simulink model "PubIfDecisionLSM_MDL"  (R2020b)
settings: configuration reference "DspaceConfig" (kept outside this file)
PostLoadFcn:
  | if any(exist('dsrtsu_mdlpostloadfcn', 'file') ~= 0), dsrtsu_mdlpostloadfcn('Execute', bdroot); end
InitFcn:
  | , if any(exist('rtifpga_mdlclblib', 'file') ~= 0), rtifpga_mdlclblib('Init', bdroot); end,
  | , if any(exist('dsmpb_private', 'file') ~= 0), dsmpb_private('dsmpb_mdlclblib', 'Init', bdroot); end,
values from neighbouring files (symbols this model uses):
  P_LSM_ALC_Enable = 0.0    [LSM_Parameter.sldd]
  P_LSM_AwayEdge_offset = 0.1    [LSM_Parameter.sldd]
  P_LSM_CentValidErr = 1.0    [LSM_Parameter.sldd]
  P_LSM_DOP_C0_EN_Limit = 0.8    [LSM_Parameter.sldd]
  P_LSM_DOP_C0_out_Limit = 2.0    [LSM_Parameter.sldd]
  P_LSM_DOP_C1_EN_Limit : value not decoded    [LSM_Parameter.sldd]
  P_LSM_DOP_C1_out_Limit : value not decoded    [LSM_Parameter.sldd]
  P_LSM_DOP_C1AndC2_Lim_X : value not decoded    [LSM_Parameter.sldd]
  P_LSM_DOP_C2_EN_Limit : value not decoded    [LSM_Parameter.sldd]
  P_LSM_DOP_C2_out_Limit : value not decoded    [LSM_Parameter.sldd]
  P_LSM_DOP_In_Pre2Dop_Dis = 1.0    [LSM_Parameter.sldd]
  P_LSM_DOP_Out_Pre2Dop_Dis = 2.0    [LSM_Parameter.sldd]
  P_LSM_DOP_PreDis_X : value not decoded    [LSM_Parameter.sldd]
  P_LSM_DOP_PreDis_Y : value not decoded    [LSM_Parameter.sldd]
  P_LSM_DOPEnableSW = 1.0    [LSM_Parameter.sldd]
  P_LSM_DOPValid_CheckTime = 0.06    [LSM_Parameter.sldd]
  P_LSM_DoubleLine_Curr2Cent_Dislimit = 0.5    [LSM_Parameter.sldd]
  P_LSM_DoubleLine_Dop2Cent_Dislimit = 0.5    [LSM_Parameter.sldd]
  P_LSM_DoubleLine_DOPOut_C1 : value not decoded    [LSM_Parameter.sldd]
  P_LSM_DoubleLine_Pre2Cent_Dislimit = 1.0    [LSM_Parameter.sldd]
  P_LSM_Error_Limit = 0.5    [LSM_Parameter.sldd]
  P_LSM_IFV2CenterAxis = 0.0    [LSM_Parameter.sldd]
  P_LSM_IFV2RearAxis = 0.0    [LSM_Parameter.sldd]
  P_LSM_Line2Edge_limit = 0.5    [LSM_Parameter.sldd]
  P_LSM_Line_Error = 0.1    [LSM_Parameter.sldd]
  P_LSM_LineSTD_Limit = 0.15    [LSM_Parameter.sldd]
  P_LSM_NOH_Switch = 0.0    [LSM_Parameter.sldd]
  P_LSM_OTL_C0_Factor = 1.0    [LSM_Parameter.sldd]
  P_LSM_OTL_C1_Factor = 0.5    [LSM_Parameter.sldd]
  P_LSM_OTL_C2_Factor = 0.5    [LSM_Parameter.sldd]
  P_LSM_Pre2OnlyLineDis = 5.0    [LSM_Parameter.sldd]
  P_LSM_Pre_t = 0.0    [LSM_Parameter.sldd]
  P_LSM_SingleLine_Cent2Edge_Dislimit = 100.0    [LSM_Parameter.sldd]
  P_LSM_SingleLine_Curr2Cent_Dislimit = 0.2    [LSM_Parameter.sldd]
  P_LSM_SingleLine_Dop2Cent_Dislimit = 0.2    [LSM_Parameter.sldd]
  P_LSM_SingleLine_DOPOut_C1 : value not decoded    [LSM_Parameter.sldd]
  P_LSM_SingleLine_Pre2Cent_Dislimit = 0.5    [LSM_Parameter.sldd]
  P_LSM_TJALimitSpd = 60.0    [LSM_Parameter.sldd]
undefined symbols (not defined in the file or in its folder): P_lCS_IFV2CenterAxis, P_LCS_IFV2RearAxis, P_LSM_EntryEdge_offset, P_LSM_EntryLnChngEnSwitch, P_LSM_EntryVanishDis, P_LSM_LinetLostTime, P_LSM_LineWijCal_C12, P_LSM_LineWijCal_C13, P_LSM_MapValid_ErrorSwitch, P_LSM_PosLineLcFac, P_LSM_SpdLim_Stub_Spd, P_LSM_SpdLim_StubLength, P_LSM_SpdTurnAlarm
libraries: simulink x324, TrueDurationTime x11
(part 12 of 25)

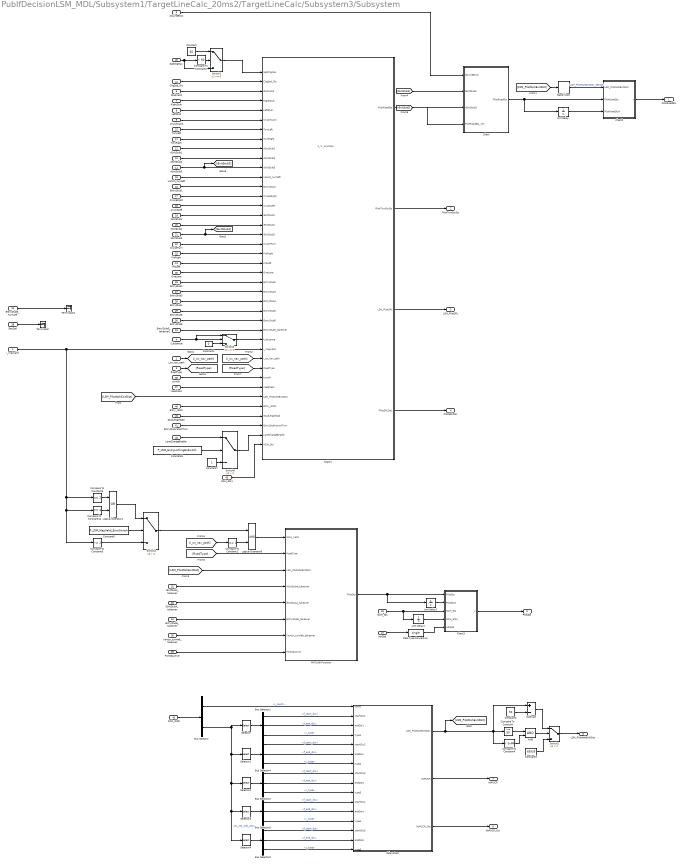
== system PubIfDecisionLSM_MDL/Subsystem1/TargetLineCalc_20ms2/TargetLineCalc/Subsystem3/Subsystem ==
  note: b_is_available
  i_mapvalid : Inport
  i_on_nav_path : Inport  Port=2
  RoadType : Inport  Port=3
  f_distance : Inport  Port=4
  bIsLineExist : Inport  Port=5
  StubValid : Inport  Port=6
  RightStub : Inport  Port=7
  LeftStub : Inport  Port=8
  CruiseValid : Inport  Port=9
  TurnLeft : Inport  Port=10
  TurnRight : Inport  Port=11
  rExitStub1 : Inport  Port=12
  rExitStub2 : Inport  Port=13
  rExitStub3 : Inport  Port=14
  Vanish_turnleft : Inport  Port=15
  EntryStub1 : Inport  Port=16
  CruiseRight : Inport  Port=17
  CruiseLeft : Inport  Port=18
  lExitStub1 : Inport  Port=19
  lExitStub2 : Inport  Port=20
  lExitStub3 : Inport  Port=21
  CruiseTurn : Inport  Port=22
  FrbRight : Inport  Port=23
  FrbLeft : Inport  Port=24
  OneLane : Inport  Port=25
  EntryStub2 : Inport  Port=26
  EntryStub3 : Inport  Port=27
  EntryStub4 : Inport  Port=28
  EntryStub5 : Inport  Port=29
  EntryStub6 : Inport  Port=30
  EntryStub5_TurnLeft : Inport  Port=31
  rExitStub4_takeover : Inport  Port=32
  lExitStub4_takeover : Inport  Port=33
  EntryStub5_takeover : Inport  Port=34
  Vanish_turnleft_takeover : Inport  Port=35
  turndir : Inport  Port=36
  roadClass : Inport  Port=37
  DecSpd : Inport  Port=38  OutDataTypeStr=uint8
  ForbidActive : Inport  Port=39
  StudLengthSpd : Inport  Port=40
  EntryStubVanishTurn : Inport  Port=41
  RFM_ODD : Inport  Port=42  OutDataTypeStr=Bus: RFM_ODD_BUS  PortDimensions=1  BusOutputAsStruct=on
  NOH_Sts : Inport  Port=43
  ChgSpd_Dis : Inport  Port=44
  SpdChgMax : Inport  Port=45
  Entry_dC0V : Inport  Port=46
  vehSpd : Inport  Port=47
  LaneChangeEnable : Inport  Port=48
  AND : Logic  AllPortsSameDT=off  OutDataTypeStr=boolean
  Bus Selector : BusSelector  OutputSignals=i_count,st_not_odd_vec
  Bus Selector{1..5} (5 alike) : BusSelector  OutputSignals=f_start_dis,f_end_dis,i_type
  Chart : Stateflow chart  TreatAsAtomicUnit=on
      settings: PortSchema="{\"entries\":[{\"content\":{\"sides\":[{\"content\":{\"connectorIds\":[\"In2\",\"In3\",\"In4\",\"In1\"]},\"type\":\"ConnectorPlacement.EquallySpacedRectSide\",\"uuid\":\"cb5dbf47-71a9-4c68-a9a0-e20b9a6c2f96\"},{\"content\":{\"connectorIds\":[\"Out1\"],\"side\":\"RIGHT\"},\"type\":\"ConnectorPlacement.EquallySpacedRectSide\",\"uuid\":\"d94cb245-01e7-4aac-95f6-b5a2c86f74a4\"},{\"content\":{\"connectorIds\":[],\"side\":\"TOP\"},\"type\":\"ConnectorPlacement.EquallySpacedRectSide\",\"uuid\":\"b16bae50-db94-4c56-a3f9-d57c33f49c97\"},{\"content\":{\"connectorIds\":[],\"side\":\"HIDDEN\"},\"type\":\"ConnectorPlacement.EquallySpacedRectSide\",\"uuid\":\"ebc0363f-4109-4233-98c7-946dda5a9c96\"}]},\"type\":\"ConnectorPlacement.EquallySpacedConnector\",\"uuid\":\"99392276-8e03-4fff-8aa1-93f14ecf3ea7\"}],\"packageUris\":[\"http://schema.mathworks.com/mf0/Connector/R2020b\"],\"version\":\"1.0\"}"
  Chart1 : Stateflow chart  TreatAsAtomicUnit=on
      settings: PortSchema="{\"entries\":[{\"content\":{\"sides\":[{\"content\":{\"connectorIds\":[\"In40\",\"In39\",\"In1\",\"In2\",\"In4\",\"In5\",\"In6\",\"In7\",\"In10\",\"In11\",\"In22\",\"In8\",\"In9\",\"In15\",\"In14\",\"In19\",\"In20\",\"In21\",\"In17\",\"In24\",\"In23\",\"In25\",\"In18\",\"In26\",\"In27\",\"In28\",\"In29\",\"In30\",\"In16\",\"In12\",\"In13\",\"In3\",\"In31\",\"In32\",\"In33\",\"In34\",\"In35\",\"In36\",\"In37\",\"In38\"]},\"type\":\"ConnectorPlacement.EquallySpacedRectSide\",\"uuid\":\"77f3efae-110f-49ea-917e-ae218e9f5cc2\"},{\"content\":{\"connectorIds\":[\"Out1\",\"Out2\",\"Out3\",\"Out4\"],\"side\":\"RIGHT\"},\"type\":\"ConnectorPlacement.EquallySpacedRectSide\",\"uuid\":\"2d94deb3-5275-495d-8df1-e01272a631f4\"},{\"content\":{\"connectorIds\":[],\"side\":\"TOP\"},\"type\":\"ConnectorPlacement.EquallySpacedRectSide\",\"uuid\":\"28314d3e-7dbf-498a-8d7e-47e3fdfafbd6\"},{\"content\":{\"connectorIds\":[],\"side\":\"HIDDEN\"},\"type\":\"ConnectorPlacement.EquallySpacedRectSide\",\"uuid\":\"3f9bf8b9-b1e2-405d-95be-6477a1260bee\"}]},\"type\":\"ConnectorPlacement.EquallySpacedConnector\",\"uuid\":\"276e7b9f-5b1f-44bf-bcdb-8855a9c8dee8\"}],\"packageUris\":[\"http://schema.mathworks.com/mf0/Connector/R2020b\"],\"version\":\"1.0\"}"
  Chart2 : Stateflow chart  TreatAsAtomicUnit=on
  Chart3 : Stateflow chart  TreatAsAtomicUnit=on
      settings: PortSchema="{\"entries\":[{\"content\":{\"sides\":[{\"content\":{\"connectorIds\":[\"In1\",\"In4\",\"In2\",\"In3\",\"In5\"]},\"type\":\"ConnectorPlacement.EquallySpacedRectSide\",\"uuid\":\"2a855711-103d-4afd-b0dc-20bc03fcd3b0\"},{\"content\":{\"connectorIds\":[\"Out1\"],\"side\":\"RIGHT\"},\"type\":\"ConnectorPlacement.EquallySpacedRectSide\",\"uuid\":\"9c6efe1d-7b4b-42ad-a8c7-d9bdd5462576\"},{\"content\":{\"connectorIds\":[],\"side\":\"TOP\"},\"type\":\"ConnectorPlacement.EquallySpacedRectSide\",\"uuid\":\"89e81c27-b573-4513-8c47-d8079b6a1114\"},{\"content\":{\"connectorIds\":[],\"side\":\"HIDDEN\"},\"type\":\"ConnectorPlacement.EquallySpacedRectSide\",\"uuid\":\"aa56bddb-9370-4270-a964-1a71b37db55c\"}]},\"type\":\"ConnectorPlacement.EquallySpacedConnector\",\"uuid\":\"d90e930b-4b5f-4761-8d41-dad0e7596f83\"}],\"packageUris\":[\"http://schema.mathworks.com/mf0/Connector/R2020b\"],\"version\":\"1.0\"}"
  Compare To Constant : simulink/Logic and Bit Operations/Compare To Constant  relop=>=  const=50  OutDataTypeStr=boolean
  Compare To Constant1 : simulink/Logic and Bit Operations/Compare To Constant  relop===  const=1  OutDataTypeStr=boolean
  Compare To Constant12 : simulink/Logic and Bit Operations/Compare To Constant  relop===  const=3  OutDataTypeStr=boolean
  Compare To Constant2 : simulink/Logic and Bit Operations/Compare To Constant  relop=<  const=60  OutDataTypeStr=boolean
  Compare To Constant4 : simulink/Logic and Bit Operations/Compare To Constant  relop=<  const=0xffff  OutDataTypeStr=boolean
  Compare To Constant5 : simulink/Logic and Bit Operations/Compare To Constant  relop===  const=2  OutDataTypeStr=boolean
  Compare To Constant6 : simulink/Logic and Bit Operations/Compare To Constant  relop=>=  const=2  OutDataTypeStr=boolean
  Constant : Constant  Value=60
  Constant2 : Constant  Value=50  OutDataTypeStr=uint16
  Constant3 : Constant  Value=65535  OutDataTypeStr=uint16
  Constant4 : Constant  Value=0  OutDataTypeStr=single
  Constant5 : Constant  Value=P_LSM_MapValid_ErrorSwitch
  Constant6 : Constant  Value=P_LSM_EntryLnChngEnSwitch
  Constant7 : Constant
  Data Type Conversion : DataTypeConversion  OutDataTypeStr=single
  EntryStub5_takeover1 : InportShadow  Port=34
  Logical Operator1 : Logic  Operator=OR  AllPortsSameDT=off  OutDataTypeStr=boolean
  Logical Operator6 : Logic  AllPortsSameDT=off  OutDataTypeStr=boolean
  MATLAB Function : MATLAB Function  TreatAsAtomicUnit=on
  NOH_Sts1 : InportShadow  Port=43
  Selector : Selector  InputPortWidth=5  IndexOptions=Index vector (dialog)  Indices=1  OutputSizes=1
  Selector1 : Selector  InputPortWidth=5  IndexOptions=Index vector (dialog)  Indices=2  OutputSizes=1
  Selector2 : Selector  InputPortWidth=5  IndexOptions=Index vector (dialog)  Indices=3  OutputSizes=1
  Selector3 : Selector  InputPortWidth=5  IndexOptions=Index vector (dialog)  Indices=4  OutputSizes=1
  Selector4 : Selector  InputPortWidth=5  IndexOptions=Index vector (dialog)  Indices=5  OutputSizes=1
  Signal Copy : SignalConversion  OverrideOpt=off
  Subsystem : Subsystem
  Subtract : Sum  Inputs=+-
  Switch1 : Switch
  Switch2 : Switch  Criteria=u2 > Threshold
  Switch3 : Switch
  Switch4 : Switch  Criteria=u2 > Threshold
  Switch6 : Switch  Criteria=u2 > Threshold
  Terminator : Terminator
  Terminator1 : Terminator
  Unit Delay : UnitDelay  SampleTime=-1  HasFrameUpgradeWarning=on
  Unit Delay1 : UnitDelay  SampleTime=-1  HasFrameUpgradeWarning=on
  Unit Delay2 : UnitDelay  SampleTime=-1  HasFrameUpgradeWarning=on
  PilotRoadSts : Outport
  PilotTurnSwSts : Outport  Port=2
  LSM_PilotSPL : Outport  Port=3
  PilotSPLDist : Outport  Port=4
  PilotSts : Outport  Port=5
  LSM_PilotNohExitDist : Outport  Port=6  OutDataTypeStr=uint16  PortDimensions=1  BusOutputAsStruct=on
  NoPUCR : Outport  Port=7
  NoPUCR_Dis : Outport  Port=8
  wires:
  ChgSpd_Dis/1 -> Chart1/39(ChgSpd_Dis)
  Switch1/1 -> Chart1/40(SpdChgMax)
  Constant/1 -> Switch1/1
  Compare To Constant2/1 -> Switch1/2
  SpdChgMax/1 -> Compare To Constant2/1, Switch1/3
  NOH_Sts1/1 -> Chart1/38(NOH_Sts)
  EntryStub5_takeover1/1 -> Chart1/30(EntryStub5_takeover)
  EntryStub5_TurnLeft/1 -> Terminator1/1
  Switch6/1 -> Chart1/37(LaneChangeEnable)
  EntryStubVanishTurn/1 -> Chart1/36(EntryStubVanishTurn)
  [RoadType] -> MATLAB Function/2(RoadType)
  [RoadType] -> Chart1/3(RoadType)
  RoadType/1 -> [RoadType]
  [i_on_nav_path] -> Compare To Constant1/1
  i_on_nav_path/1 -> [i_on_nav_path]
  Constant7/1 -> Switch6/3
  LaneChangeEnable/1 -> Switch6/1
  Constant6/1 -> Switch6/2
  Compare To Constant6/1 -> Switch4/3
  Switch4/1 -> Logical Operator6/1
  Constant5/1 -> Switch4/2
  Logical Operator1/1 -> Switch4/1
  Compare To Constant5/1 -> Logical Operator1/1
  Switch3/1 -> Chart1/16(f_distance)
  Constant4/1 -> Switch3/3
  Data Type Conversion/1 -> Chart3/5(vehSpd)
  Chart3/1(y) -> PilotSts/1
  StudLengthSpd/1 -> Chart1/35(StudLengthSpd)
  vehSpd/1 -> Data Type Conversion/1
  Unit Delay2/1 -> Chart3/4(PilotStsK)
  ForbidActive/1 -> MATLAB Function/8(ForbidActive)
  DecSpd/1 -> Terminator/1
  Subsystem/2(NoPUCR) -> NoPUCR/1
  Subsystem/3(NoPUCR_Dis) -> NoPUCR_Dis/1
  roadClass/1 -> Chart1/32(roadClass)
  Subsystem/1(LSM_PilotNohExitDist) -> [LSM_PilotNohExitDist], Compare To Constant4/1, Compare To Constant/1, Subtract/1
  Bus Selector3/3 -> Subsystem/16(type5)  "<i_type>"
  Bus Selector3/2 -> Subsystem/15(endDis5)  "<f_end_dis>"
  Bus Selector3/1 -> Subsystem/14(startDis5)  "<f_start_dis>"
  Bus Selector5/3 -> Subsystem/13(type4)  "<i_type>"
  Bus Selector5/2 -> Subsystem/12(endDis4)  "<f_end_dis>"
  Bus Selector5/1 -> Subsystem/11(startDis4)  "<f_start_dis>"
  Selector3/1 -> Bus Selector5/1
  Bus Selector2/3 -> Subsystem/10(type3)  "<i_type>"
  Bus Selector2/2 -> Subsystem/9(endDis3)  "<f_end_dis>"
  Bus Selector2/1 -> Subsystem/8(startDis3)  "<f_start_dis>"
  Bus Selector4/3 -> Subsystem/7(type2)  "<i_type>"
  Bus Selector4/2 -> Subsystem/6(endDis2)  "<f_end_dis>"
  Bus Selector1/3 -> Subsystem/4(type1)  "<i_type>"
  Bus Selector4/1 -> Subsystem/5(startDis2)  "<f_start_dis>"
  Bus Selector1/2 -> Subsystem/3(endDis1)  "<f_end_dis>"
  Bus Selector1/1 -> Subsystem/2(startDis1)  "<f_start_dis>"
  Bus Selector/1 -> Subsystem/1(count)  "<i_count>"
  Selector1/1 -> Bus Selector4/1
  Selector4/1 -> Bus Selector3/1
  Selector2/1 -> Bus Selector2/1
  Selector/1 -> Bus Selector1/1
  Bus Selector/2 -> Selector/1, Selector1/1, Selector2/1, Selector3/1, Selector4/1  "<st_not_odd_vec>"
  RFM_ODD/1 -> Bus Selector/1
  turndir/1 -> Chart1/31(turndir)
  f_distance/1 -> Switch3/2, Switch3/1
  Vanish_turnleft_takeover/1 -> MATLAB Function/7(Vanish_turnleft_takeover)
  EntryStub5_takeover/1 -> MATLAB Function/6(EntryStub5_takeover)
  lExitStub4_takeover/1 -> MATLAB Function/5(lExitStub4_takeover)
  rExitStub4_takeover/1 -> MATLAB Function/4(rExitStub4_takeover)
  i_mapvalid/1 -> Compare To Constant5/1, Compare To Constant6/1, Compare To Constant12/1, Chart1/12(i_mapvalid)
  Logical Operator6/1 -> MATLAB Function/1(NOH_Valid)
  MATLAB Function/1(PilotSts) -> Unit Delay2/1, Chart3/1(PilotSts)
  Compare To Constant1/1 -> Logical Operator6/2
  Compare To Constant12/1 -> Logical Operator1/2
  EntryStub2/1 -> Chart1/18(EntryStub2)
  [i_on_nav_path] -> Chart1/13(i_on_nav_path)
  lExitStub2/1 -> Chart1/20(lExitStub2)
  TurnRight/1 -> Chart1/7(TurnRight)
  rExitStub3/1 -> Chart1/22(rExitStub3), [rExitStub3]
  Chart1/4(PilotSPLDist) -> PilotSPLDist/1
  CruiseTurn/1 -> Chart1/17(CruiseTurn)
  StubValid/1 -> Chart1/1(StubValid)
  CruiseLeft/1 -> Chart1/14(CruiseLeft)
  EntryStub4/1 -> Chart1/27(EntryStub4)
  EntryStub3/1 -> Chart1/26(EntryStub3)
  OneLane/1 -> Chart1/25(OneLane)
  FrbLeft/1 -> Chart1/23(FrbLeft)
  CruiseRight/1 -> Chart1/15(CruiseRight)
  Vanish_turnleft/1 -> Chart1/8(Vanish_turnleft)
  LeftStub/1 -> Chart1/4(LeftStub)
  RightStub/1 -> Chart1/2(RightStub)
  lExitStub1/1 -> Chart1/19(lExitStub1)
  EntryStub6/1 -> Chart1/29(EntryStub6)
  bIsLineExist/1 -> Chart/2(bIsLineExist)
  CruiseValid/1 -> Chart1/5(CruiseValid)
  rExitStub1/1 -> Chart1/10(rExitStub1)
  Chart/1(PilotRoadSts) -> Chart2/2(PilotRoadSts), Unit Delay/1
  EntryStub1/1 -> Chart1/9(EntryStub1)
  rExitStub2/1 -> Chart1/11(rExitStub2)
  TurnLeft/1 -> Chart1/6(TurnLeft)
  [lExitStub3] -> Chart/3(lExitStub3)
  Chart1/1(PilotRoadSts) -> Chart/1(PilotRoadSts_init)
  FrbRight/1 -> Chart1/24(FrbRight)
  EntryStub5/1 -> Chart1/28(EntryStub5)
  lExitStub3/1 -> Chart1/21(lExitStub3), [lExitStub3]
  [rExitStub3] -> Chart/4(rExitStub3)
  Chart1/2(PilotTurnSwSts) -> PilotTurnSwSts/1
  [LSM_PilotNohExitDist] -> Chart1/33(LSM_PilotNohExitDist)
  Chart2/1(y) -> PilotRoadSts/1
  Unit Delay/1 -> Chart2/3(PilotRoadStsK)
  [LSM_PilotNohExitDist] -> Signal Copy/1
  Signal Copy/1 -> Chart2/1(LSM_PilotNohExitDist)  "LSM_PilotNohExitDist_Set100"
  NOH_Sts/1 -> Unit Delay1/1, Chart3/2(NOH_Sts)
  Unit Delay1/1 -> Chart3/3(NOH_StsK)
  [LSM_PilotNohExitDist] -> MATLAB Function/3(LSM_PilotNohExitDist)
  Entry_dC0V/1 -> Chart1/34(Entry_dC0V)
  Chart1/3(LSM_PilotSPL) -> LSM_PilotSPL/1
  Constant2/1 -> Subtract/2
  Switch2/1 -> LSM_PilotNohExitDist/1
  Compare To Constant/1 -> AND/1
  Subtract/1 -> Switch2/1
  Constant3/1 -> Switch2/3
  Compare To Constant4/1 -> AND/2
  AND/1 -> Switch2/2

== system PubIfDecisionLSM_MDL/Subsystem1/TargetLineCalc_20ms2/TargetLineCalc/Subsystem3/Subsystem1 ==
  i_mapvalid : Inport
  i_on_nav_path : Inport  Port=2
  RoadType : Inport  Port=3
  NoPUCR : Inport  Port=4
  f_distance : Inport  Port=5
  MATLAB Function : MATLAB Function  TreatAsAtomicUnit=on
  Subsystem : Subsystem
  Unit Delay{,1..9} (10 alike) : UnitDelay  SampleTime=-1  HasFrameUpgradeWarning=on
  i_mapvalid_out : Outport
  i_on_nav_path_out : Outport  Port=2
  RoadType_out : Outport  Port=3
  wires:
  NoPUCR/1 -> Subsystem/2(NoPUCR)
  MATLAB Function/3(RoadType_out) -> RoadType_out/1
  Unit Delay9/1 -> MATLAB Function/7(f_distanceK)
  Unit Delay8/1 -> MATLAB Function/6(RoadTypeK)
  Unit Delay6/1 -> MATLAB Function/4(i_on_nav_pathK)
  Unit Delay5/1 -> MATLAB Function/2(i_mapvalidK)
  i_mapvalid/1 -> MATLAB Function/1(i_mapvalid), Unit Delay5/1
  RoadType/1 -> MATLAB Function/5(RoadType), Unit Delay8/1
  i_on_nav_path/1 -> MATLAB Function/3(i_on_nav_path), Unit Delay6/1
  f_distance/1 -> Unit Delay9/1
  Unit Delay/1 -> MATLAB Function/12(i_on_nav_path_storeK)
  MATLAB Function/6(RoadStore) -> Unit Delay2/1
  MATLAB Function/4(count) -> Unit Delay4/1
  Unit Delay1/1 -> MATLAB Function/11(i_mapvalid_storeK)
  Unit Delay4/1 -> MATLAB Function/8(countK)
  MATLAB Function/5(time_trigger) -> Unit Delay3/1
  Unit Delay2/1 -> MATLAB Function/10(RoadStoreK)
  MATLAB Function/7(i_mapvalid_store) -> Unit Delay1/1
  Unit Delay3/1 -> MATLAB Function/9(timing_triggerK)
  MATLAB Function/9(f_distance_store) -> Unit Delay7/1
  Unit Delay7/1 -> MATLAB Function/13(f_distance_storeK)
  MATLAB Function/8(i_on_nav_path_store) -> Unit Delay/1
  MATLAB Function/1(i_mapvalid_out) -> i_mapvalid_out/1
  MATLAB Function/2(i_on_nav_path_out) -> Subsystem/1(u)
  Subsystem/1(y) -> i_on_nav_path_out/1
